simulink model "pid_test"  (R2020b)
settings: Solver=FixedStepDiscrete  StartTime=0.0  StopTime=10  FixedStep=0.001  RelTol=1e-3
values from neighbouring files (symbols this model uses):
  B = 0.0003    [demo.m]    (also in motor.m; param_motor.mat; pendulo_modelo.m)
  J = (M+m)*r^2    (= 1.5e-05)    [demo.m]    (also in motor.m; param_motor.mat; pendulo_modelo.m)
  Kb = 0.0308    [demo.m]    (also in motor.m; param_motor.mat; pendulo_modelo.m)
  Kp = 0.0494    [demo.m]    (also in motor.m; param_motor.mat; pendulo_modelo.m)
  L = 0.0105    [motor.m]    (also in param_motor.mat)
  M = 0.1    [demo.m]    (also in motor.m; param_motor.mat; pendulo_modelo.m)
  m = 0.5    [demo.m]    (also in motor.m; param_motor.mat; pendulo_modelo.m)
  r = 0.005    [demo.m]    (also in motor.m; param_motor.mat; pendulo_modelo.m)
  R = 0.005    [demo.m]    (also in motor.m = 6.84; param_motor.mat = 6.84; pendulo_modelo.m)
libraries: pid_lib x1
settings Model: Creator=aleca  LastModifiedBy=aleca

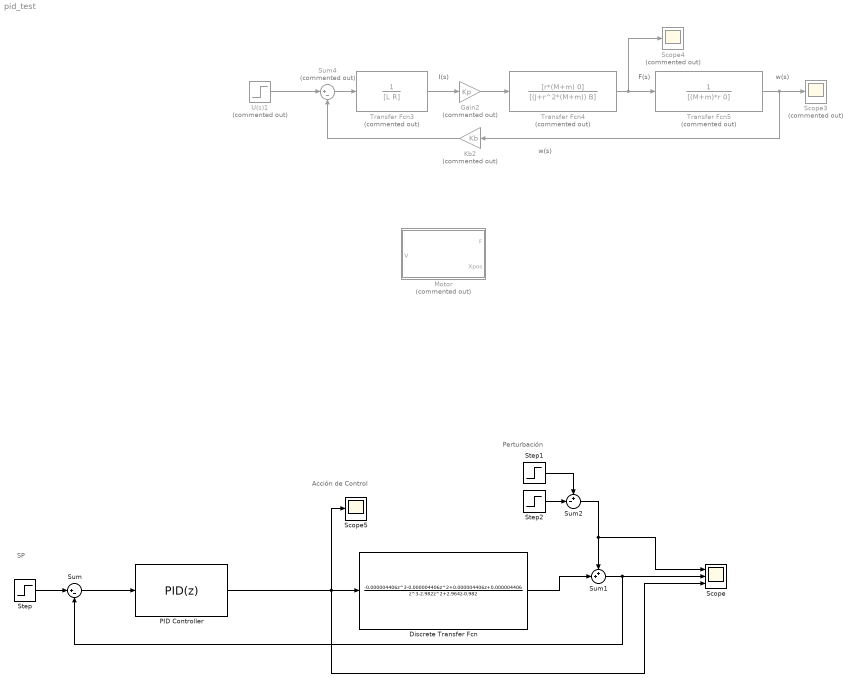
== system pid_test ==
  note: Acción de Control
  note: SP
  note: Perturbación
  note: F(s)
  note: w(s)
  note: I(s)
  note: w(s)
  Discrete Transfer Fcn : DiscreteTransferFcn  Numerator=[-0.000004406 -0.000004406 0.000004406 0.000004406]  Denominator=[1 -2.982 2.964 -0.982]
  Gain2 : Gain  Commented=on  Gain=Kp
  Kb2 : Gain  Commented=on  Gain=Kb
  Motor : Subsystem  Commented=on
  PID Controller : pid_lib/PID Controller  Controller=PID  Form=Parallel  TimeDomain=Discrete-time  UseExternalTs=off  SampleTime=-1  IntegratorMethod=Forward Euler  FilterMethod=Forward Euler  ControllerParametersSource=internal  P=-45.105963300228  I=-190.380002129331  D=-1.61573367788201  UseFilter=on  N=167.531798593719  TunerSelectOption=Transfer Function Based (PID Tuner App)  InitialConditionSource=internal  InitialConditionForIntegrator=0  InitialConditionForFilter=0  DifferentiatorICPrevScaledInput=0  ExternalReset=none  TrackingMode=off  Kt=1  LimitOutput=off  SatLimitsSource=internal  UpperSaturationLimit=inf  LowerSaturationLimit=-inf  LinearizeAsGain=on  AntiWindupMode=none  Kb=1  POutMin=[]  POutMax=[]  IOutMin=[]  IOutMax=[]  DOutMin=[]  DOutMax=[]  NOutMin=[]  NOutMax=[]  SumOutMin=[]  SumOutMax=[]  SaturationOutMin=[]  SaturationOutMax=[]  PParamMin=[]  PParamMax=[]  IParamMin=[]  IParamMax=[]  DParamMin=[]  DParamMax=[]  NParamMin=[]  NParamMax=[]  KbParamMin=[]  KbParamMax=[]  KtParamMin=[]  KtParamMax=[]  KbOutMin=[]  KbOutMax=[]  KtOutMin=[]  KtOutMax=[]  IntegratorOutMin=[]  IntegratorOutMax=[]  FilterOutMin=[]  FilterOutMax=[]  SumI1OutMin=[]  SumI1OutMax=[]  SumI2OutMin=[]  SumI2OutMax=[]  SumI3OutMin=[]  SumI3OutMax=[]  SumI4OutMin=[]  SumI4OutMax=[]  SumDOutMin=[]  SumDOutMax=[]  DifferentiatorOutMin=[]  DifferentiatorOutMax=[]  FilterDiffOutCoefMin=[]  FilterDiffOutCoefMax=[]  ReciprocalOutMin=[]  ReciprocalOutMax=[]  SumDenOutMin=[]  SumDenOutMax=[]  SumNumOutMin=[]  SumNumOutMax=[]  DivideOutMin=[]  DivideOutMax=[]  UdiffTsProdOutMin=[]  UdiffTsProdOutMax=[]  NTsProdOutMin=[]  NTsProdOutMax=[]  UintegralTsProdOutMin=[]  UintegralTsProdOutMax=[]  UngainTsProdOutMin=[]  UngainTsProdOutMax=[]  IntegratorContinuousStateAttributes=''  IntegratorStateMustResolveToSignalObject=off  IntegratorRTWStateStorageClass=Auto  FilterContinuousStateAttributes=''  FilterStateMustResolveToSignalObject=off  FilterRTWStateStorageClass=Auto  ParallelPVariant=InternalParameters  IdealPVariant=Disabled  IVariant=InternalParameters  DVariant=InternalParameters  IntegratorVariant=Discrete  SatVariant=Disabled  AWVariant=Passthrough  PCopyVariant=Disabled  TRVariant=Disabled  FdbkBlocksVariant=Forward  IdealPFdbkVariant=Disabled  SatFdbkVariant=Disabled  DerivativeFilterVariant=ForwardEulerFilter  NVariant=InternalParameters  NCopyVariant=Disabled  FilterICVariant=InternalICsFilter  IntegratorICVariant=InternalICs  ExternalResetVariant=Disabled  TRSumVariant=Passthrough  SumFdbkVariant=Disabled  SumVariant=Sum_PID  TsampFilterVariant=InternalTs  TsampNgainVariant=Passthrough  TsampIntegralVariant=Passthrough  ExternalSaturationOutDataTypeStr=Inherit: Same as second input
  Scope : Scope  NumInputPorts=3
  Scope3 : Scope  Commented=on
  Scope4 : Scope  Commented=on
  Scope5 : Scope
  Step : Step  After=0  SampleTime=0
  Step1 : Step  Time=3  After=0.08
  Step2 : Step  Time=3.1  After=0.08  SampleTime=0
  Sum : Sum  Inputs=|+-
  Sum1 : Sum  Inputs=++|
  Sum2 : Sum  Inputs=+-|
  Sum4 : Sum  Commented=on  Inputs=|+-
  Transfer Fcn3 : TransferFcn  Commented=on  Denominator=[L R]
  Transfer Fcn4 : TransferFcn  Commented=on  Numerator=[r*(M+m) 0]  Denominator=[(J+r^2*(M+m)) B]
  Transfer Fcn5 : TransferFcn  Commented=on  Denominator=[(M+m)*r 0]
  U(s)1 : Step  Commented=on  After=12  SampleTime=0
  wires:
  Step/1 -> Sum/1
  Discrete Transfer Fcn/1 -> Sum1/2
  Sum1/1 -> Sum/2, Scope/2
  Sum4/1 -> Transfer Fcn3/1
  Gain2/1 -> Transfer Fcn4/1
  U(s)1/1 -> Sum4/1
  Transfer Fcn3/1 -> Gain2/1
  Kb2/1 -> Sum4/2
  Transfer Fcn5/1 -> Kb2/1, Scope3/1
  Transfer Fcn4/1 -> Scope4/1, Transfer Fcn5/1
  PID Controller/1 -> Discrete Transfer Fcn/1, Scope5/1, Scope/3
  Sum/1 -> PID Controller/1
  Step1/1 -> Sum2/1
  Step2/1 -> Sum2/2
  Sum2/1 -> Sum1/1, Scope/1

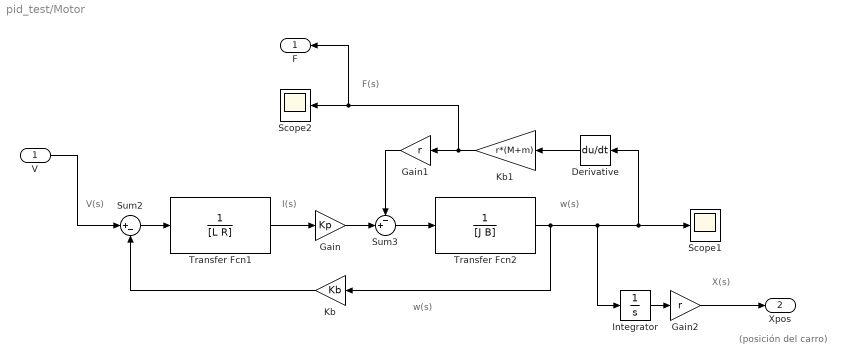
== system pid_test/Motor ==
  note: (posición del carro)
  note: w(s)
  note: F(s)
  note: I(s)
  note: w(s)
  note: X(s)
  note: V(s)
  V : Inport
  Derivative : Derivative
  Gain : Gain  Gain=Kp
  Gain1 : Gain  Gain=r
  Gain2 : Gain  Gain=r
  Integrator : Integrator
  Kb : Gain  Gain=Kb
  Kb1 : Gain  Gain=r*(M+m)
  Scope1 : Scope
  Scope2 : Scope
  Sum2 : Sum  Inputs=|+-
  Sum3 : Sum  Inputs=-+|
  Transfer Fcn1 : TransferFcn  Denominator=[L R]
  Transfer Fcn2 : TransferFcn  Denominator=[J B]
  F : Outport
  Xpos : Outport  Port=2
  wires:
  Gain1/1 -> Sum3/1
  Transfer Fcn2/1 -> Kb/1, Integrator/1, Scope1/1, Derivative/1
  Gain/1 -> Sum3/2
  Kb/1 -> Sum2/2
  Kb1/1 -> F/1, Scope2/1, Gain1/1
  Transfer Fcn1/1 -> Gain/1
  Sum2/1 -> Transfer Fcn1/1
  Sum3/1 -> Transfer Fcn2/1
  Derivative/1 -> Kb1/1
  V/1 -> Sum2/1
  Integrator/1 -> Gain2/1
  Gain2/1 -> Xpos/1
